simulink library "dac18"  (Simulink 7.5)
settings: Solver=ode45  SolverMode=SingleTasking  StartTime=0.0  StopTime=10.0  RelTol=1e-3
settings Model: Creator=rolf  LastModifiedBy=controls

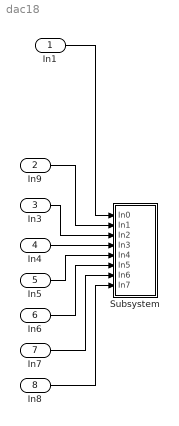
== system dac18 ==
  In1 : Inport  OutDataType=sfix(16)  OutScaling=2^0
  In9 : Inport  Port=2  OutDataType=sfix(16)  OutScaling=2^0
  In3 : Inport  Port=3  OutDataType=sfix(16)  OutScaling=2^0
  In4 : Inport  Port=4  OutDataType=sfix(16)  OutScaling=2^0
  In5 : Inport  Port=5  OutDataType=sfix(16)  OutScaling=2^0
  In6 : Inport  Port=6  OutDataType=sfix(16)  OutScaling=2^0
  In7 : Inport  Port=7  OutDataType=sfix(16)  OutScaling=2^0
  In8 : Inport  Port=8  OutDataType=sfix(16)  OutScaling=2^0
  Subsystem : Subsystem
  wires:
  In1/1 -> Subsystem/1(In0)
  In3/1 -> Subsystem/3(In2)
  In4/1 -> Subsystem/4(In3)
  In5/1 -> Subsystem/5(In4)
  In6/1 -> Subsystem/6(In5)
  In7/1 -> Subsystem/7(In6)
  In8/1 -> Subsystem/8(In7)
  In9/1 -> Subsystem/2(In1)

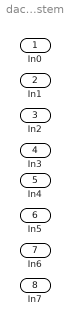
== system dac18/Subsystem ==
  In0 : Inport  OutDataType=sfix(16)  OutScaling=2^0
  In1 : Inport  Port=2  OutDataType=sfix(16)  OutScaling=2^0
  In2 : Inport  Port=3  OutDataType=sfix(16)  OutScaling=2^0
  In3 : Inport  Port=4  OutDataType=sfix(16)  OutScaling=2^0
  In4 : Inport  Port=5  OutDataType=sfix(16)  OutScaling=2^0
  In5 : Inport  Port=6  OutDataType=sfix(16)  OutScaling=2^0
  In6 : Inport  Port=7  OutDataType=sfix(16)  OutScaling=2^0
  In7 : Inport  Port=8  OutDataType=sfix(16)  OutScaling=2^0
